simulink model "SpeedManager"  (R2023b)
settings: Solver=VariableStepAuto  StartTime=0.0  StopTime=10.0  RelTol=1e-3
settings Model: Creator=monis  LastModifiedBy=monis

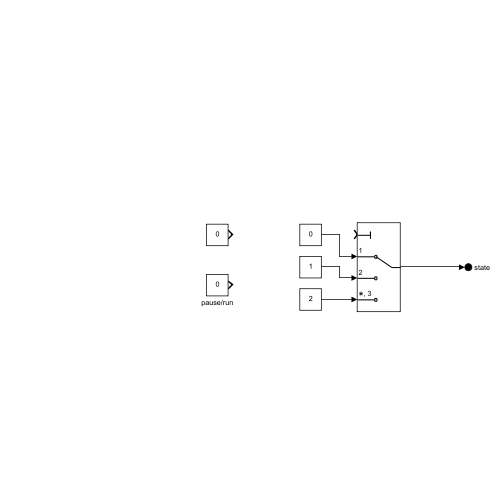
[thumbnail: Simulink's stored preview of the top-level diagram]
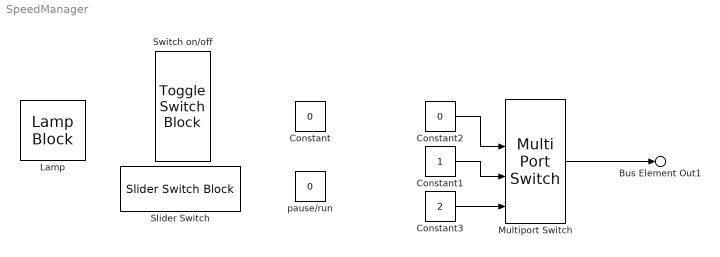
== system SpeedManager ==
  Constant : Constant  Value=0
  Constant1 : Constant
  Constant2 : Constant  Value=0
  Constant3 : Constant  Value=2
  Lamp : LampBlock  LabelPosition=Hide
  Multiport Switch : MultiPortSwitch  DataPortOrder=Specify indices  SaturateOnIntegerOverflow=off  InputSameDT=off
  Slider Switch : SliderSwitchBlock
      settings: Values={{'Off', 'On'}, [0 1]}
  Switch on/off : ToggleSwitchBlock
      settings: Values={{'Off', 'On'}, [0 1]}
  pause/run : Constant  Value=0
  Bus Element Out1 : Outport  PortName=state
  wires:
  Multiport Switch/1 -> Bus Element Out1/1
  Constant3/1 -> Multiport Switch/4
  Constant1/1 -> Multiport Switch/3
  Constant2/1 -> Multiport Switch/2
